simulink model "untitled"  (R2023a)
settings: Solver=VariableStepAuto  StartTime=0.0  StopTime=4/frecuency  RelTol=1e-3
undefined symbols (not defined in the file): C, frecuency, L, R, Vs
libraries: spsFourierLib x8, spsSeriesRLCBranchLib x7, spsMultimeterLib x2, spsACVoltageSourceLib x2, spsCurrentMeasurementLib x1, sps_lib x1
settings Model: Creator=USUARIO  LastModifiedBy=Juan Esteban

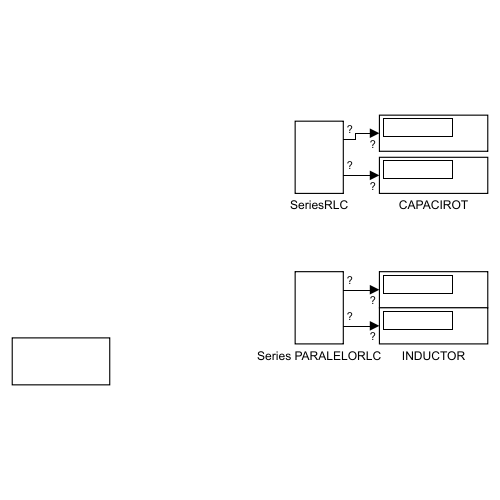
[thumbnail: Simulink's stored preview of the top-level diagram]
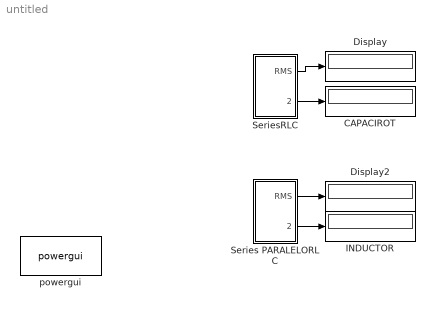
== system untitled ==
  CAPACIROT : Display
  Display : Display
  Display2 : Display
  INDUCTOR : Display
  Series PARALELORLC : Subsystem
  SeriesRLC : Subsystem
  powergui : sps_lib/powergui  Priority=1  SimulationMode=Continuous  SampleTime=50e-6  frequency=60  Iterations=50  frequencyindice=5004.87242427344  Pbase=100e6  ErrMax=1e-4  UnitsV=kV  UnitsW=MW  buscounter=0  FunctionMessages=off  echomessages=off  EnableUseOfTLC=off  CurrentSourceSwitches=off  DisableSnubberDevices=off  DisableRonSwitches=off  DisableVfSwitches=off  DisplayEquations=off  AutomaticDiscreteSolvers=off  SolverType=Tustin/Backward Euler (TBE)  Interpol=off  ExternalGateDelay=off  methode=off  Ts=100  x0status=blocks  SPID=on  SwTol=0  HookPort=off  NonlinearTolerance=1e-4  nMaxIteration=100  ContinueOnMaxIteration=off  RestoreLinks=warning  ResistiveCurrentMeasurement=off  Frange=[0:2:500]  Ylog=off  Xlog=on  ShowGrid=off  save=off  variable=ZData  structure=0  ZoomFFT=off  StartTime=0.0  cycles=1  DisplayStyle=1  fundamental=60  FreqAxis=off  MaxFrequency=1000  frequencyindicesteady=1  RmsSteady=1  display=off
  wires:
  SeriesRLC/1(RMS) -> Display/1
  SeriesRLC/2(Phasor) -> CAPACIROT/1
  Series PARALELORLC/1(RMS) -> Display2/1
  Series PARALELORLC/2(Phasor) -> INDUCTOR/1

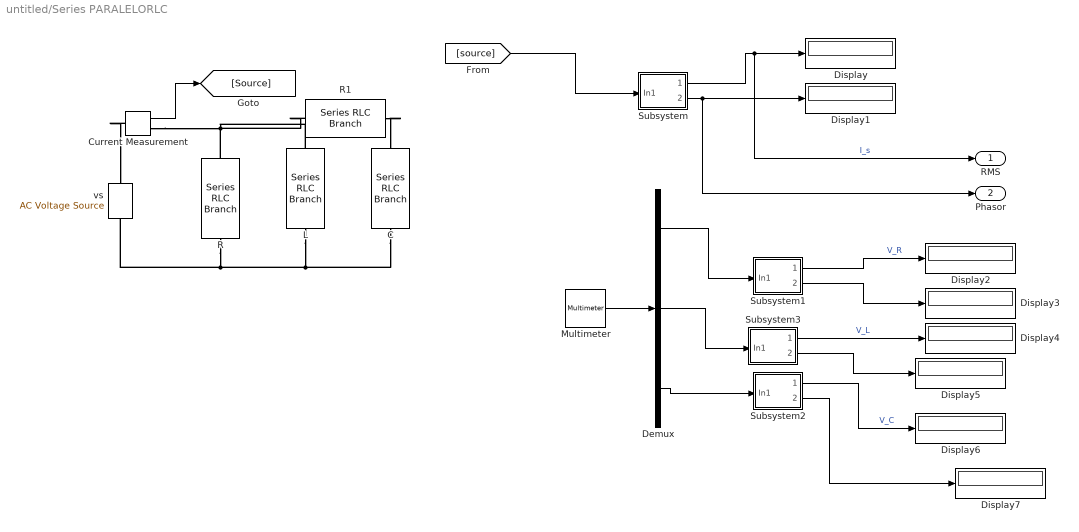
== system untitled/Series PARALELORLC ==
  C : spsSeriesRLCBranchLib/Series RLC Branch  LConnTagsString=__new0  RConnTagsString=__new0  BranchType=C  Resistance=1  Inductance=1e-3  SetiL0=off  InitialCurrent=0  Capacitance=C  Setx0=off  InitialVoltage=0  Measurements=Branch voltage and current
  Current Measurement : spsCurrentMeasurementLib/Current Measurement  PhasorSimulation=off  OutputType=Complex  PSBequivalent=0
  Demux : Demux  Outputs=3
  Display{,1..7} (8 alike) : Display
  L : spsSeriesRLCBranchLib/Series RLC Branch  LConnTagsString=__new0  RConnTagsString=__new0  BranchType=L  Resistance=1  Inductance=L  SetiL0=off  InitialCurrent=0  Capacitance=1e-6  Setx0=off  InitialVoltage=0  Measurements=Branch voltage and current
  Multimeter : spsMultimeterLib/Multimeter  L=11  sel=1  yselected={}  Gain=0  OutputType=Complex  PlotAtSimulationStop=off  PhasorSimulation=off
  R : spsSeriesRLCBranchLib/Series RLC Branch  LConnTagsString=__new0  RConnTagsString=__new0  BranchType=R  Resistance=R  Inductance=1e-3  SetiL0=off  InitialCurrent=0  Capacitance=1e-6  Setx0=off  InitialVoltage=0  Measurements=Branch current
  R1 : spsSeriesRLCBranchLib/Series RLC Branch  LConnTagsString=__new0  RConnTagsString=__new0  BranchType=R  Resistance=1e-4  Inductance=1e-3  SetiL0=off  InitialCurrent=0  Capacitance=1e-6  Setx0=off  InitialVoltage=0  Measurements=Branch voltage and current
  Subsystem : Subsystem
  Subsystem1 : Subsystem
  Subsystem2 : Subsystem
  Subsystem3 : Subsystem
  vs : spsACVoltageSourceLib/AC Voltage Source  Amplitude=Vs*sqrt(2)  Phase=0  Frequency=frecuency  SampleTime=0  Measurements=None  BusType=swing  Pref=10e3  Qref=0  Qmin=-inf  Qmax=+inf
  RMS : Outport
  Phasor : Outport  Port=2
  wires:
  Subsystem2/2(Phasor) -> Display7/1
  Subsystem1/1(RMS) -> Display2/1  "V_R"
  Subsystem2/1(RMS) -> Display6/1  "V_C"
  Subsystem3/1(RMS) -> Display4/1  "V_L"
  Multimeter/1 -> Demux/1
  Subsystem3/2(Phasor) -> Display5/1
  Subsystem/2(Phasor) -> Phasor/1, Display1/1
  Demux/3 -> Subsystem2/1(In1)
  Subsystem1/2(Phasor) -> Display3/1
  Subsystem/1(RMS) -> RMS/1, Display/1  "I_s"
  Current Measurement/1 -> [Source]
  [source] -> Subsystem/1(In1)
  Demux/1 -> Subsystem1/1(In1)
  Demux/2 -> Subsystem3/1(In1)
  connections:
  C/RConn1 -- R/RConn1 -- vs/LConn1 -- L/LConn1
  R/LConn1 -- R1/RConn1 -- L/RConn1 -- Current Measurement/RConn1
  Current Measurement/LConn1 -- vs/RConn1
  R1/LConn1 -- C/LConn1

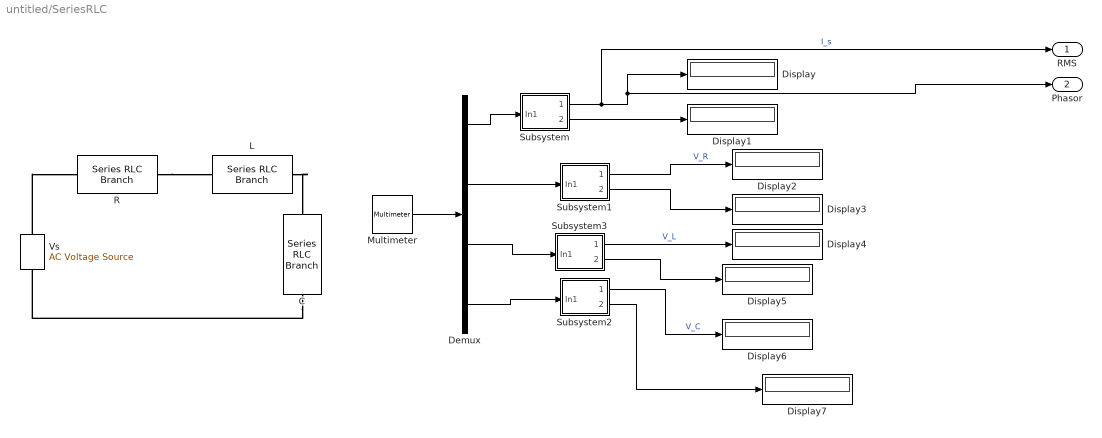
== system untitled/SeriesRLC ==
  C : spsSeriesRLCBranchLib/Series RLC Branch  LConnTagsString=__new0  RConnTagsString=__new0  BranchType=C  Resistance=1  Inductance=1e-3  SetiL0=off  InitialCurrent=0  Capacitance=C  Setx0=off  InitialVoltage=0  Measurements=Branch voltage
  Demux : Demux
  Display{,1..7} (8 alike) : Display
  L : spsSeriesRLCBranchLib/Series RLC Branch  LConnTagsString=__new0  RConnTagsString=__new0  BranchType=L  Resistance=1  Inductance=L  SetiL0=off  InitialCurrent=0  Capacitance=1e-6  Setx0=off  InitialVoltage=0  Measurements=Branch voltage
  Multimeter : spsMultimeterLib/Multimeter  L=11  sel=[11 6 5 4]  yselected={}  Gain=[1 1 1 1]  OutputType=Complex  PlotAtSimulationStop=off  PhasorSimulation=off
  R : spsSeriesRLCBranchLib/Series RLC Branch  LConnTagsString=__new0  RConnTagsString=__new0  BranchType=R  Resistance=R  Inductance=1e-3  SetiL0=off  InitialCurrent=0  Capacitance=1e-6  Setx0=off  InitialVoltage=0  Measurements=Branch voltage and current
  Subsystem : Subsystem
  Subsystem1 : Subsystem
  Subsystem2 : Subsystem
  Subsystem3 : Subsystem
  Vs : spsACVoltageSourceLib/AC Voltage Source  Amplitude=Vs*sqrt(2)  Phase=0  Frequency=frecuency  SampleTime=0  Measurements=None  BusType=swing  Pref=10e3  Qref=0  Qmin=-inf  Qmax=+inf
  RMS : Outport
  Phasor : Outport  Port=2
  wires:
  Demux/1 -> Subsystem/1(In1)
  Demux/2 -> Subsystem1/1(In1)
  Demux/3 -> Subsystem3/1(In1)
  Demux/4 -> Subsystem2/1(In1)
  Subsystem/2(Phasor) -> Display1/1
  Subsystem1/1(RMS) -> Display2/1  "V_R"
  Subsystem1/2(Phasor) -> Display3/1
  Subsystem3/1(RMS) -> Display4/1  "V_L"
  Subsystem3/2(Phasor) -> Display5/1
  Subsystem2/1(RMS) -> Display6/1  "V_C"
  Subsystem2/2(Phasor) -> Display7/1
  Multimeter/1 -> Demux/1
  Subsystem/1(RMS) -> RMS/1, Phasor/1, Display/1  "I_s"
  connections:
  R/RConn1 -- L/RConn1
  L/LConn1 -- C/LConn1
  C/RConn1 -- Vs/LConn1
  Vs/RConn1 -- R/LConn1

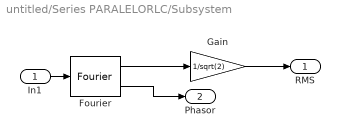
== system untitled/Series PARALELORLC/Subsystem ==
  In1 : Inport
  Fourier : spsFourierLib/Fourier  Freq=frecuency  n=1  InInit=[0, 0]  Ts=0
  Gain : Gain  Gain=1/sqrt(2)
  RMS : Outport
  Phasor : Outport  Port=2
  wires:
  In1/1 -> Fourier/1
  Fourier/1 -> Gain/1
  Fourier/2 -> Phasor/1
  Gain/1 -> RMS/1

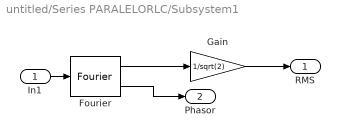
== system untitled/Series PARALELORLC/Subsystem1 ==
  In1 : Inport
  Fourier : spsFourierLib/Fourier  Freq=frecuency  n=1  InInit=[0, 0]  Ts=0
  Gain : Gain  Gain=1/sqrt(2)
  RMS : Outport
  Phasor : Outport  Port=2
  wires:
  In1/1 -> Fourier/1
  Fourier/1 -> Gain/1
  Fourier/2 -> Phasor/1
  Gain/1 -> RMS/1

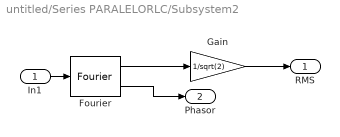
== system untitled/Series PARALELORLC/Subsystem2 ==
  In1 : Inport
  Fourier : spsFourierLib/Fourier  Freq=frecuency  n=1  InInit=[0, 0]  Ts=0
  Gain : Gain  Gain=1/sqrt(2)
  RMS : Outport
  Phasor : Outport  Port=2
  wires:
  In1/1 -> Fourier/1
  Fourier/1 -> Gain/1
  Fourier/2 -> Phasor/1
  Gain/1 -> RMS/1

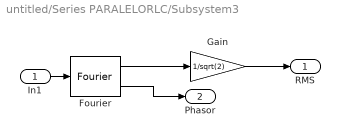
== system untitled/Series PARALELORLC/Subsystem3 ==
  In1 : Inport
  Fourier : spsFourierLib/Fourier  Freq=frecuency  n=1  InInit=[0, 0]  Ts=0
  Gain : Gain  Gain=1/sqrt(2)
  RMS : Outport
  Phasor : Outport  Port=2
  wires:
  In1/1 -> Fourier/1
  Fourier/1 -> Gain/1
  Fourier/2 -> Phasor/1
  Gain/1 -> RMS/1

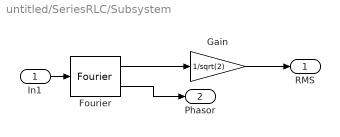
== system untitled/SeriesRLC/Subsystem ==
  In1 : Inport
  Fourier : spsFourierLib/Fourier  Freq=frecuency  n=1  InInit=[0, 0]  Ts=0
  Gain : Gain  Gain=1/sqrt(2)
  RMS : Outport
  Phasor : Outport  Port=2
  wires:
  In1/1 -> Fourier/1
  Fourier/1 -> Gain/1
  Fourier/2 -> Phasor/1
  Gain/1 -> RMS/1

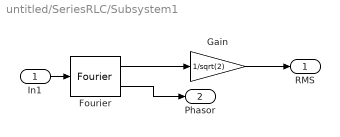
== system untitled/SeriesRLC/Subsystem1 ==
  In1 : Inport
  Fourier : spsFourierLib/Fourier  Freq=frecuency  n=1  InInit=[0, 0]  Ts=0
  Gain : Gain  Gain=1/sqrt(2)
  RMS : Outport
  Phasor : Outport  Port=2
  wires:
  In1/1 -> Fourier/1
  Fourier/1 -> Gain/1
  Fourier/2 -> Phasor/1
  Gain/1 -> RMS/1

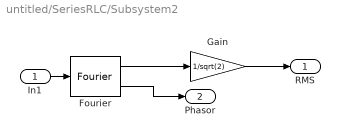
== system untitled/SeriesRLC/Subsystem2 ==
  In1 : Inport
  Fourier : spsFourierLib/Fourier  Freq=frecuency  n=1  InInit=[0, 0]  Ts=0
  Gain : Gain  Gain=1/sqrt(2)
  RMS : Outport
  Phasor : Outport  Port=2
  wires:
  In1/1 -> Fourier/1
  Fourier/1 -> Gain/1
  Fourier/2 -> Phasor/1
  Gain/1 -> RMS/1

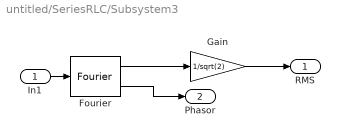
== system untitled/SeriesRLC/Subsystem3 ==
  In1 : Inport
  Fourier : spsFourierLib/Fourier  Freq=frecuency  n=1  InInit=[0, 0]  Ts=0
  Gain : Gain  Gain=1/sqrt(2)
  RMS : Outport
  Phasor : Outport  Port=2
  wires:
  In1/1 -> Fourier/1
  Fourier/1 -> Gain/1
  Fourier/2 -> Phasor/1
  Gain/1 -> RMS/1
